simulink model "Lab_3"  (R2025b)
settings: Solver=VariableStepAuto  StartTime=0.0  StopTime=4200  RelTol=1e-3
values from neighbouring files (symbols this model uses):
  K1 = 10 / 400    (= 0.025)    [Lab1_3.m]
  K2 = 400 / 230    (= 1.73913043478)    [Lab1_3.m]
  tau = 10 * 60    (= 600)    [Lab1_3.m]
  u_aus = -0.75    [Lab1_3.m]
  u_ein = 0.75    [Lab1_3.m]
settings Model: Creator=rishabh  LastModifiedBy=rishabh

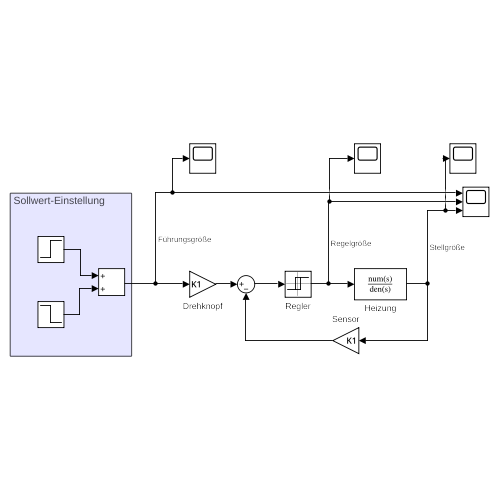
[thumbnail: Simulink's stored preview of the top-level diagram]
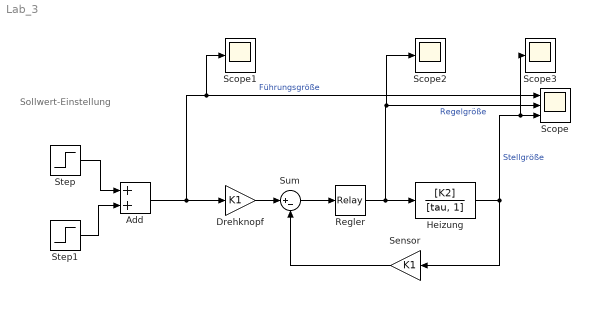
== system Lab_3 ==
  note: Sollwert-Einstellung
  Add : Sum
  Drehknopf : Gain  Gain=K1
  Heizung : TransferFcn  Numerator=[K2]  Denominator=[tau, 1]
  Regler : Relay  OnSwitchValue=u_ein  OffSwitchValue=u_aus  OnOutputValue=230
  Scope : Scope  NumInputPorts=3
      settings: ActiveDisplayYMinimum=-28.749999999999993  ActiveDisplayYMaximum=258.75  YLabel=Temperatur in °C
  Scope1 : Scope
      settings: ActiveDisplayYMinimum=-28.749999999999993  ActiveDisplayYMaximum=258.75  YLabel=Temperatur in °C
  Scope2 : Scope
      settings: ActiveDisplayYMinimum=-28.749999999999993  ActiveDisplayYMaximum=258.75  YLabel=Temperatur in °C  DataLoggingVariableName=ScopeData2
  Scope3 : Scope
      settings: ActiveDisplayYMinimum=-28.749999999999993  ActiveDisplayYMaximum=258.75  YLabel=Temperatur in °C  DataLoggingVariableName=ScopeData3
  Sensor : Gain  Gain=K1
  Step : Step  Time=0  After=180  SampleTime=0
  Step1 : Step  Time=1800  After=-180  SampleTime=0
  Sum : Sum  Inputs=|+-
  wires:
  Drehknopf/1 -> Sum/1
  Sum/1 -> Regler/1
  Regler/1 -> Scope2/1, Scope/2, Heizung/1  "Regelgröße"
  Heizung/1 -> Sensor/1, Scope3/1, Scope/3  "Stellgröße"
  Sensor/1 -> Sum/2
  Step/1 -> Add/1
  Step1/1 -> Add/2
  Add/1 -> Scope1/1, Scope/1, Drehknopf/1  "Führungsgröße"
